simulink model "assignment1DEPRECATED"  (R2023b)
settings: Solver=FixedStepAuto  StartTime=0.0  StopTime=5  FixedStep=1e-3  RelTol=1e-3  EnableMultiTasking=on
undefined symbols (not defined in the file): D0, D1, D10, D11, D12, D13, D2, D3, D4, D5, D6, D7, D8, D9, PTA0, PTA1, PTA2, PTB23, PTB9, PTC16, PTC17, PTC2, PTC3, PTC4, PTD0, PTD1, PTD2, PTD3
libraries: frdmk64flib x18, dspstat3 x3
settings Model: PacingRate=2  ExtModeTrigDuration=5  Creator=Nicholas  LastModifiedBy=Nicholas
settings OptimizationCC: EnhancedBackFolding=on  PassReuseOutputArgsAs=Individual arguments  ZeroExternalMemoryAtStartup=off  ZeroInternalMemoryAtStartup=off  MaxStackSize=64  OptimizeBlockOrder=speed  DifferentSizesBufferReuse=on  OptimizationCustomize=off  EfficientTunableParamExpr=on
settings DebuggingCC: ParameterTunabilityLossMsg=error
settings HardwareCC: ProdBitPerPointer=32  ProdBitPerSizeT=32  ProdBitPerPtrDiffT=32  ProdLargestAtomicInteger=Long  ProdLargestAtomicFloat=Double  ProdWordSize=32  ProdHWDeviceType=ARM Compatible->ARM Cortex
settings SFSimCC: MATLABDynamicMemAlloc=off
settings RTWCC: Description=Embedded Coder  SystemTargetFile=ert.tlc  HardwareBoard=NXP FRDM-K64F  TLCOptions="-aInlineSetEventsForThisBaseRateFcn=TLC_FALSE -aSuppressMultiTaskScheduler=TLC_FALSE  -aRateBasedStepFcn=0"  TemplateMakefile=ert_default_tmf  Toolchain=GNU Tools for ARM Embedded Processors
settings CodeAppCC: ForceParamTrailComments=on  IgnoreCustomStorageClasses=off  OperatorAnnotations=on  SimulinkDataObjDesc=on  SFDataObjDesc=on  InsertBlockDesc=on
settings ERTTargetCC: ExtModeTransport=4  ExtModeMexFile=sendToCommService

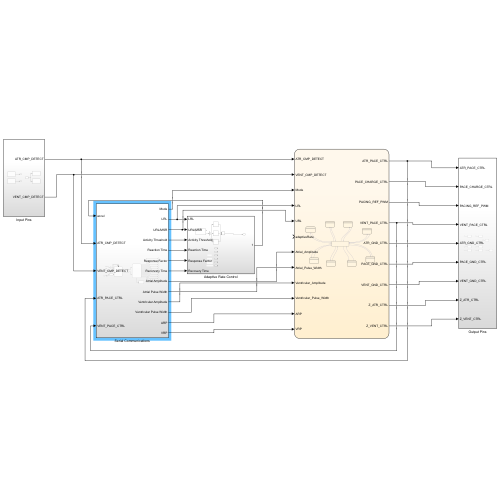
[thumbnail: Simulink's stored preview of the top-level diagram]
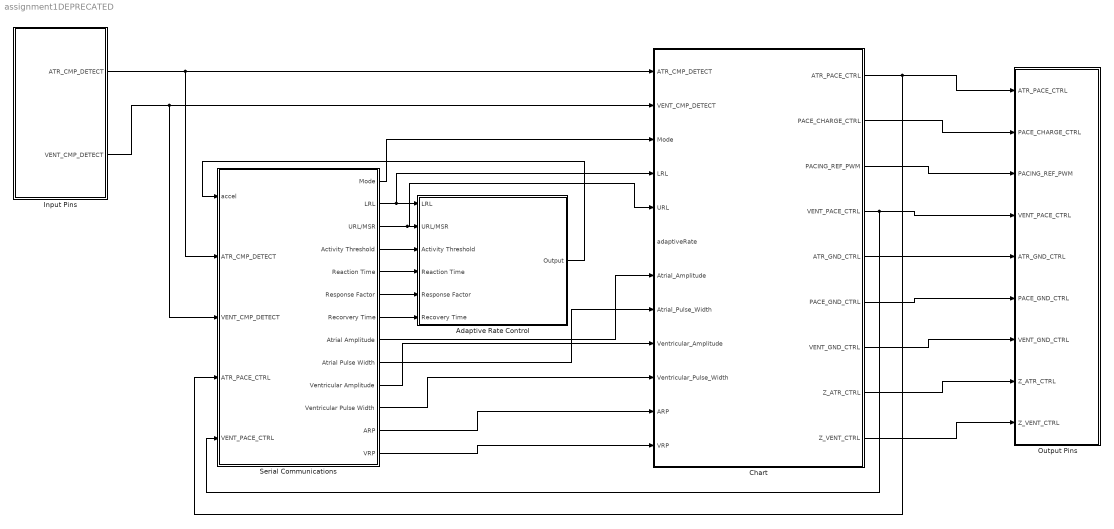
== system assignment1DEPRECATED ==
  Adaptive Rate Control : Subsystem
  Chart : Stateflow chart  TreatAsAtomicUnit=on
      settings: PortSchema="{\"entries\":[{\"content\":{\"sides\":[{\"content\":{\"connectorIds\":[\"In1\",\"In2\",\"In3\",\"In11\",\"In10\",\"In12\",\"In4\",\"In5\",\"In6\",\"In7\",\"In8\",\"In9\"]},\"type\":\"ConnectorPlacement.EquallySpacedRectSide\",\"uuid\":\"f4000909-515d-4a0d-a478-4ca4207159b3\"},{\"content\":{\"connectorIds\":[\"Out1\",\"Out2\",\"Out3\",\"Out4\",\"Out5\",\"Out6\",\"Out7\",\"Out8\",\"Out9\"],\"side\":\"RIGHT\"},\"type\":\"ConnectorPlacement.EquallySpacedRectSide\",\"uuid\":\"74c20bfd-42d0-453a-b20e-355357afff28\"},{\"content\":{\"side\":\"TOP\"},\"type\":\"ConnectorPlacement.EquallySpacedRectSide\",\"uuid\":\"0265984b-474f-4dc0-b8ea-569a4f78f123\"}]},\"type\":\"ConnectorPlacement.EquallySpacedConnector\",\"uuid\":\"44478604-183f-4c3e-8da1-5539e792ac80\"}],\"packageUris\":[\"http://schema.mathworks.com/mf0/Connector/R2020b\"],\"version\":\"1.0\"}"
  Input Pins : Subsystem  Description=Maps the digital and analog input pins of the K64F to named variables as defined in Pacemaker Shield Explained
  Output Pins : Subsystem
  Serial Communications : Subsystem
  wires:
  Input Pins/1(ATR_CMP_DETECT) -> Serial Communications/2(ATR_CMP_DETECT), Chart/1(ATR_CMP_DETECT)
  Input Pins/2(VENT_CMP_DETECT) -> Serial Communications/3(VENT_CMP_DETECT), Chart/2(VENT_CMP_DETECT)
  Chart/9(Z_VENT_CTRL) -> Output Pins/9(Z_VENT_CTRL)
  Chart/4(VENT_PACE_CTRL) -> Serial Communications/5(VENT_PACE_CTRL), Output Pins/4(VENT_PACE_CTRL)
  Chart/8(Z_ATR_CTRL) -> Output Pins/8(Z_ATR_CTRL)
  Chart/3(PACING_REF_PWM) -> Output Pins/3(PACING_REF_PWM)
  Chart/1(ATR_PACE_CTRL) -> Serial Communications/4(ATR_PACE_CTRL), Output Pins/1(ATR_PACE_CTRL)
  Chart/2(PACE_CHARGE_CTRL) -> Output Pins/2(PACE_CHARGE_CTRL)
  Chart/6(PACE_GND_CTRL) -> Output Pins/6(PACE_GND_CTRL)
  Chart/5(ATR_GND_CTRL) -> Output Pins/5(ATR_GND_CTRL)
  Chart/7(VENT_GND_CTRL) -> Output Pins/7(VENT_GND_CTRL)
  Serial Communications/3(URL/MSR) -> Chart/10(URL), Adaptive Rate Control/2(URL/MSR)
  Serial Communications/2(LRL) -> Chart/11(LRL), Adaptive Rate Control/1(LRL)
  Serial Communications/1(Mode) -> Chart/3(Mode)
  Serial Communications/8(Atrial Amplitude) -> Chart/4(Atrial_Amplitude)
  Serial Communications/10(Ventricular Amplitude) -> Chart/6(Ventricular_Amplitude)
  Serial Communications/9(Atrial Pulse Width) -> Chart/5(Atrial_Pulse_Width)
  Serial Communications/11(Ventricular Pulse Width) -> Chart/7(Ventricular_Pulse_Width)
  Serial Communications/13(VRP) -> Chart/9(VRP)
  Serial Communications/12(ARP) -> Chart/8(ARP)
  Adaptive Rate Control/1(Output) -> Serial Communications/1(accel)
  Serial Communications/4(Activity Threshold) -> Adaptive Rate Control/3(Activity Threshold)
  Serial Communications/6(Response Factor) -> Adaptive Rate Control/5(Response Factor)
  Serial Communications/5(Reaction Time) -> Adaptive Rate Control/4(Reaction Time)
  Serial Communications/7(Recorvery Time) -> Adaptive Rate Control/6(Recovery Time)

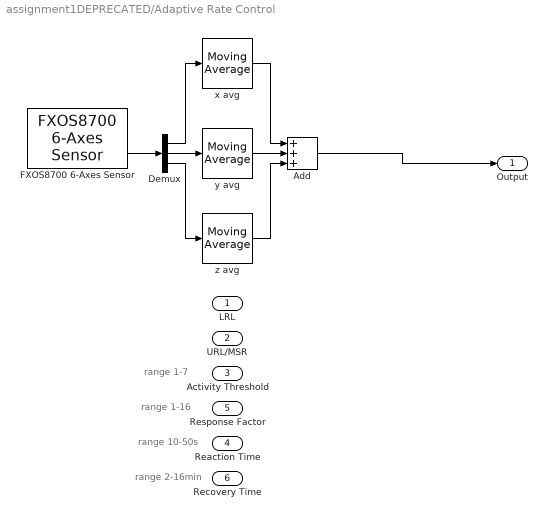
== system assignment1DEPRECATED/Adaptive Rate Control ==
  note: range 2-16min
  note: range 1-16
  note: range 10-50s
  note: range 1-7
  LRL : Inport
  URL/MSR : Inport  Port=2
  Activity Threshold : Inport  Port=3
  Reaction Time : Inport  Port=4
  Response Factor : Inport  Port=5
  Recovery Time : Inport  Port=6
  Add : Sum  Inputs=+++
  Demux : Demux  Outputs=3
  FXOS8700 6-Axes Sensor : frdmk64flib/FXOS8700 6-Axes Sensor  Activesensor=Accelerometer and Magnetometer  ODR=100Hz  HybridODR=400Hz  Accelfullrange=-4g to +4g  SampleTime=-1
  x avg : dspstat3/Moving Average  Method=Sliding window  ForgettingFactorPort=off  SpecifyWindowLength=on  WindowLength=4  OverlapLength=3  AllowArbitraryInputLength=off  ForgettingFactor=0.9  SimulateUsing=Code generation
  y avg : dspstat3/Moving Average  Method=Sliding window  ForgettingFactorPort=off  SpecifyWindowLength=on  WindowLength=4  OverlapLength=3  AllowArbitraryInputLength=off  ForgettingFactor=0.9  SimulateUsing=Code generation
  z avg : dspstat3/Moving Average  Method=Sliding window  ForgettingFactorPort=off  SpecifyWindowLength=on  WindowLength=4  OverlapLength=3  AllowArbitraryInputLength=off  ForgettingFactor=0.9  SimulateUsing=Code generation
  Output : Outport
  wires:
  FXOS8700 6-Axes Sensor/2 -> Demux/1
  Demux/1 -> x avg/1
  Demux/2 -> y avg/1
  Demux/3 -> z avg/1
  x avg/1 -> Add/1
  y avg/1 -> Add/2
  z avg/1 -> Add/3
  Add/1 -> Output/1

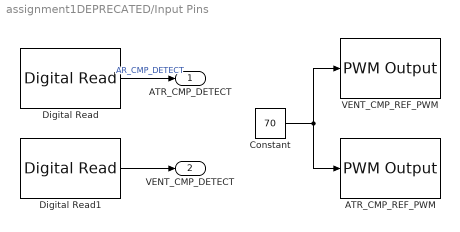
== system assignment1DEPRECATED/Input Pins ==
  ATR_CMP_REF_PWM : frdmk64flib/PWM Output  Whichpin=PTC2 (D6)  InitialFrequency=2000  InitialDutyCycle=0
  Constant : Constant  Value=70
  Digital Read : frdmk64flib/Digital Read  Whichpin=PTC16 (D0)  SampleTime=-1
  Digital Read1 : frdmk64flib/Digital Read  Whichpin=PTC17 (D1)  SampleTime=-1
  VENT_CMP_REF_PWM : frdmk64flib/PWM Output  Whichpin=PTA1 (D3)  InitialFrequency=2000  InitialDutyCycle=0
  ATR_CMP_DETECT : Outport
  VENT_CMP_DETECT : Outport  Port=2
  wires:
  Digital Read1/1 -> VENT_CMP_DETECT/1
  Digital Read/1 -> ATR_CMP_DETECT/1  "AR_CMP_DETECT"
  Constant/1 -> ATR_CMP_REF_PWM/1, VENT_CMP_REF_PWM/1

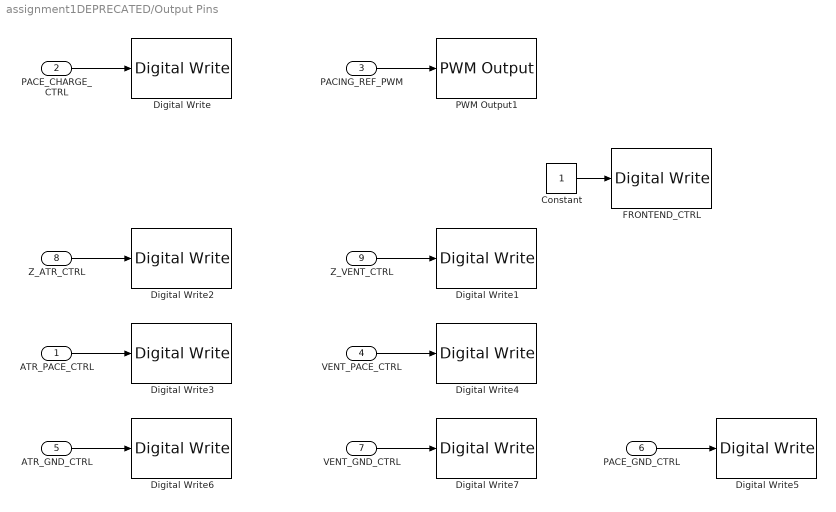
== system assignment1DEPRECATED/Output Pins ==
  ATR_PACE_CTRL : Inport
  PACE_CHARGE_CTRL : Inport  Port=2
  PACING_REF_PWM : Inport  Port=3
  VENT_PACE_CTRL : Inport  Port=4
  ATR_GND_CTRL : Inport  Port=5
  PACE_GND_CTRL : Inport  Port=6
  VENT_GND_CTRL : Inport  Port=7
  Z_ATR_CTRL : Inport  Port=8
  Z_VENT_CTRL : Inport  Port=9
  Constant : Constant
  Digital Write : frdmk64flib/Digital Write  Whichpin=PTB9 (D2)
  Digital Write1 : frdmk64flib/Digital Write  Whichpin=PTC3 (D7)
  Digital Write2 : frdmk64flib/Digital Write  Whichpin=PTB23 (D4)
  Digital Write3 : frdmk64flib/Digital Write  Whichpin=PTA0 (D8)
  Digital Write4 : frdmk64flib/Digital Write  Whichpin=PTC4 (D9)
  Digital Write5 : frdmk64flib/Digital Write  Whichpin=PTD0 (D10)
  Digital Write6 : frdmk64flib/Digital Write  Whichpin=PTD2 (D11)
  Digital Write7 : frdmk64flib/Digital Write  Whichpin=PTD3 (D12)
  FRONTEND_CTRL : frdmk64flib/Digital Write  Whichpin=PTD1 (D13)
  PWM Output1 : frdmk64flib/PWM Output  Whichpin=PTA2 (D5)  InitialFrequency=2000  InitialDutyCycle=0
  wires:
  PACE_CHARGE_CTRL/1 -> Digital Write/1
  Z_ATR_CTRL/1 -> Digital Write2/1
  PACING_REF_PWM/1 -> PWM Output1/1
  Z_VENT_CTRL/1 -> Digital Write1/1
  ATR_PACE_CTRL/1 -> Digital Write3/1
  VENT_PACE_CTRL/1 -> Digital Write4/1
  PACE_GND_CTRL/1 -> Digital Write5/1
  ATR_GND_CTRL/1 -> Digital Write6/1
  VENT_GND_CTRL/1 -> Digital Write7/1
  Constant/1 -> FRONTEND_CTRL/1

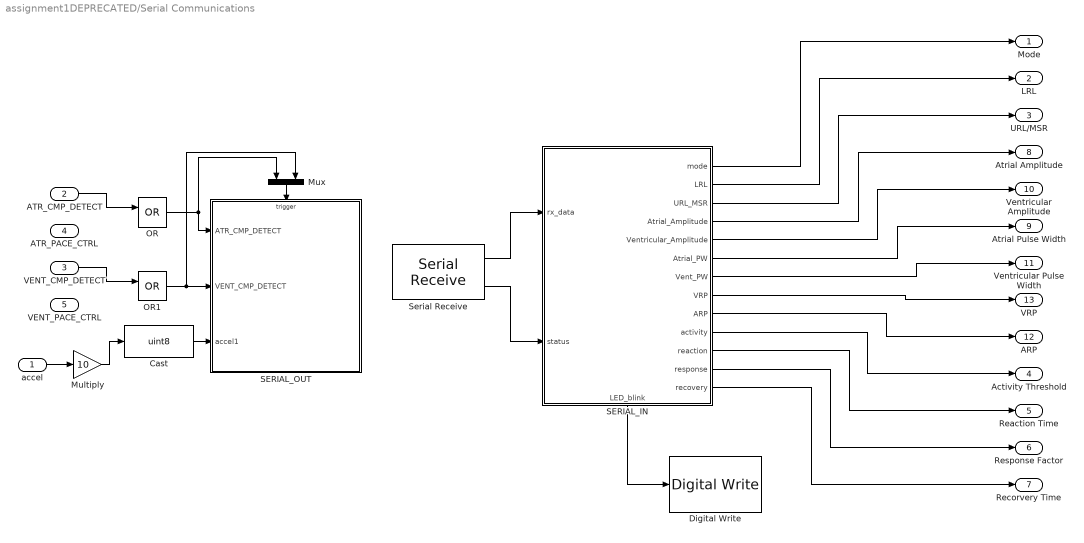
== system assignment1DEPRECATED/Serial Communications ==
  accel : Inport
  ATR_CMP_DETECT : Inport  Port=2
  VENT_CMP_DETECT : Inport  Port=3
  ATR_PACE_CTRL : Inport  Port=4
  VENT_PACE_CTRL : Inport  Port=5
  Cast : DataTypeConversion  OutDataTypeStr=uint8  SaturateOnIntegerOverflow=off  RndMeth=Floor
  Digital Write : frdmk64flib/Digital Write  Whichpin=RED_LED
  Multiply : Gain  Gain=10
  Mux : Mux  Inputs=2
  OR : Logic  Operator=OR  IconShape=distinctive  AllPortsSameDT=off  OutDataTypeStr=boolean
  OR1 : Logic  Operator=OR  IconShape=distinctive  AllPortsSameDT=off  OutDataTypeStr=boolean
  SERIAL_IN : Stateflow chart  TreatAsAtomicUnit=on
      settings: PortSchema="{\"entries\":[{\"content\":{\"sides\":[{\"content\":{\"connectorIds\":[\"In1\",\"In2\"]},\"type\":\"ConnectorPlacement.EquallySpacedRectSide\",\"uuid\":\"ebf63f13-cff1-4dfd-8253-a37fed9b5330\"},{\"content\":{\"connectorIds\":[\"Out1\",\"Out3\",\"Out2\",\"Out5\",\"Out13\",\"Out4\",\"Out7\",\"Out8\",\"Out6\",\"Out9\",\"Out10\",\"Out12\",\"Out11\"],\"side\":\"RIGHT\"},\"type\":\"ConnectorPlacement.EquallySpacedRectSide\",\"uuid\":\"8941ae37-13b3-448c-8772-44937e4639cd\"},{\"content\":{\"side\":\"TOP\"},\"type\":\"ConnectorPlacement.EquallySpacedRectSide\",\"uuid\":\"7a479970-9298-4bcf-8741-da85a2b03343\"},{\"content\":{\"connectorIds\":[\"Out14\"],\"side\":\"BOTTOM\"},\"type\":\"ConnectorPlacement.EquallySpacedRectSide\",\"uuid\":\"dbdb6486-bc4b-4aff-855d-c7d246fcadd5\"}]},\"type\":\"ConnectorPlacement.EquallySpacedConnector\",\"uuid\":\"673a7430-fbb7-42ed-bf30-7a03e16fbc4d\"}],\"packageUris\":[\"http://schema.mathworks.com/mf0/Connector/R2020b\"],\"version\":\"1.0\"}"
  SERIAL_OUT : Subsystem
  Serial Receive : frdmk64flib/Serial Receive  SCIModule=0  Baudrate=uint32(9600)  Parity=None  StopBits=1  HardwareFlowControl=None  ByteOrder=LittleEndian  DataType=uint8  DataLength=16  BlockingMode=off  OutputStatus=on  SampleTime=-1
  Mode : Outport
  LRL : Outport  Port=2
  URL/MSR : Outport  Port=3
  Activity Threshold : Outport  Port=4
  Reaction Time : Outport  Port=5
  Response Factor : Outport  Port=6
  Recorvery Time : Outport  Port=7
  Atrial Amplitude : Outport  Port=8
  Atrial Pulse Width : Outport  Port=9
  Ventricular Amplitude : Outport  Port=10
  Ventricular Pulse Width : Outport  Port=11
  ARP : Outport  Port=12
  VRP : Outport  Port=13
  wires:
  Serial Receive/2 -> SERIAL_IN/2(status)
  Serial Receive/1 -> SERIAL_IN/1(rx_data)
  SERIAL_IN/1(mode) -> Mode/1
  SERIAL_IN/3(LRL) -> LRL/1
  SERIAL_IN/2(URL_MSR) -> URL/MSR/1
  SERIAL_IN/5(Atrial_Amplitude) -> Atrial Amplitude/1
  SERIAL_IN/4(Atrial_PW) -> Atrial Pulse Width/1
  SERIAL_IN/6(ARP) -> ARP/1
  SERIAL_IN/7(Vent_PW) -> Ventricular Pulse Width/1
  SERIAL_IN/8(VRP) -> VRP/1
  SERIAL_IN/9(activity) -> Activity Threshold/1
  SERIAL_IN/10(reaction) -> Reaction Time/1
  SERIAL_IN/11(recovery) -> Recorvery Time/1
  SERIAL_IN/12(response) -> Response Factor/1
  SERIAL_IN/13(Ventricular_Amplitude) -> Ventricular Amplitude/1
  Mux/1 -> SERIAL_OUT/Trigger
  accel/1 -> Multiply/1
  ATR_CMP_DETECT/1 -> OR/1
  VENT_CMP_DETECT/1 -> OR1/1
  OR/1 -> SERIAL_OUT/1(ATR_CMP_DETECT), Mux/1
  OR1/1 -> SERIAL_OUT/2(VENT_CMP_DETECT), Mux/2
  SERIAL_IN/14(LED_blink) -> Digital Write/1
  Multiply/1 -> Cast/1
  Cast/1 -> SERIAL_OUT/3(accel1)

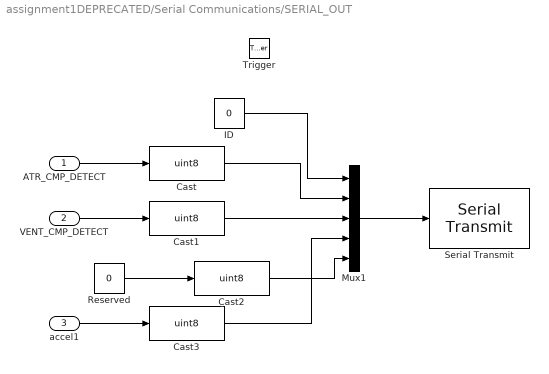
== system assignment1DEPRECATED/Serial Communications/SERIAL_OUT ==
  ATR_CMP_DETECT : Inport
  VENT_CMP_DETECT : Inport  Port=2
  accel1 : Inport  Port=3
  Trigger : TriggerPort  VariantControl=(inherit)  PortDimensions=1
  Cast{,1..3} (4 alike) : DataTypeConversion  OutDataTypeStr=uint8  SaturateOnIntegerOverflow=off  RndMeth=Floor
  ID : Constant  Value=0  OutDataTypeStr=uint8
  Mux1 : Mux  Inputs=5
  Reserved : Constant  Value=0
  Serial Transmit : frdmk64flib/Serial Transmit  SCIModule=0  Baudrate=uint32(9600)  Parity=None  StopBits=1  HardwareFlowControl=None  ByteOrder=LittleEndian  BlockingMode=on  OutputStatus=off
  wires:
  VENT_CMP_DETECT/1 -> Cast1/1
  Cast1/1 -> Mux1/3
  Cast3/1 -> Mux1/4
  Cast/1 -> Mux1/2
  accel1/1 -> Cast3/1
  ID/1 -> Mux1/1
  Reserved/1 -> Cast2/1
  Mux1/1 -> Serial Transmit/1
  ATR_CMP_DETECT/1 -> Cast/1
  Cast2/1 -> Mux1/5

== stateflow chart assignment1DEPRECATED/Serial Communications/SERIAL_IN ==
  state success
    entry:
    LED_blink = 1;
    mode = rx_data(1);
    LRL = rx_data(2);
    URL_MSR = rx_data(3);
    Atrial_Amplitude = double(rx_data(4)/10);
    Ventricular_Amplitude = double(rx_data(5)/10);
    Atrial_PW = rx_data(6);
    Vent_PW = rx_data(7);
    VRP = uint32(rx_data(8)*10);
    ARP = uint32(rx_data(9)*10);
    activity = rx_data(10);
    reaction = rx_data(11);
    response = rx_data(12);
    recovery = rx_data(13);
  state Initial
    entry:
    mode = 255;
  state standby
    entry:
    LED_blink = 0;
  (default) -> Initial
  success -> standby : [et(sec) >= 1]
  standby -> success : [status == 0]
  Initial -> standby
  data: rx_data input; status input; mode output uint8; URL_MSR output; LRL output; Atrial_PW output; Atrial_Amplitude output double; ARP output uint32; Vent_PW output; VRP output uint32; activity output; reaction output; recovery output; response output; Ventricular_Amplitude output double; LED_blink output

== stateflow chart assignment1DEPRECATED/Chart ==
  state VOO
    state setup
      entry:
      ventDutyCycle = (Ventricular_Amplitude/5)*100
      ventWait = single(Rate_ms - Ventricular_Pulse_Width)
    state charge_discharge
      entry:
      %discharge c21
      PACE_GND_CTRL = 0
      VENT_PACE_CTRL = 0
      Z_ATR_CTRL = 0
      Z_VENT_CTRL = 0
      ATR_PACE_CTRL = 0
      ATR_GND_CTRL = 0
      VENT_GND_CTRL = 1
      %charge c22
      VENT_PACE_CTRL = 0
      ATR_PACE_CTRL = 0
      PACING_REF_PWM = double(ventDutyCycle)
      PACE_CHARGE_CTRL = 1
    state pace
      PACE_CHARGE_CTRL = 0
      PACE_GND_CTRL = 1
      ATR_PACE_CTRL = 0
      ATR_GND_CTRL = 0
      Z_ATR_CTRL = 0
      Z_VENT_CTRL = 0
      VENT_GND_CTRL = 0
      VENT_PACE_CTRL = 1
    (default) -> VOO.setup
    VOO.setup -> VOO.charge_discharge
    VOO.charge_discharge -> VOO.pace : [et(msec) >= ventWait]
    VOO.pace -> VOO.charge_discharge : [et(msec) >= Ventricular_Pulse_Width]
  state AAI
    state setup
      entry:
      atrialDutyCycle = (Atrial_Amplitude/5)*100
      atrWait = single(Rate_ms - Atrial_Pulse_Width)
      timeToPace = atrWait
    state refractory_period
    state charge_discharge_EN
      entry:
      %discharge c21
      PACE_GND_CTRL = 0
      ATR_PACE_CTRL = 0
      Z_ATR_CTRL = 0
      Z_VENT_CTRL = 0
      VENT_PACE_CTRL = 0
      VENT_GND_CTRL = 0
      ATR_GND_CTRL = 1
      %charge c22
      ATR_PACE_CTRL = 0
      VENT_PACE_CTRL = 0
      PACING_REF_PWM = atrialDutyCycle
      PACE_CHARGE_CTRL = 1
    state sense_wait
      exit:
      timeToPace = timeToPace - et(msec)
    state pace
      entry:
      PACE_CHARGE_CTRL = 0
      PACE_GND_CTRL = 1
      VENT_PACE_CTRL = 0
      VENT_GND_CTRL = 0
      Z_ATR_CTRL = 0
      Z_VENT_CTRL = 0
      ATR_GND_CTRL = 0
      ATR_PACE_CTRL = 1
      %reset timer
      timeToPace = atrWait
    (default) -> AAI.setup
    AAI.setup -> AAI.charge_discharge_EN
    AAI.refractory_period -> AAI.sense_wait : [et(msec) >= ARP]
    AAI.sense_wait -> AAI.refractory_period [order 1] : [ATR_CMP_DETECT == 1]
    AAI.charge_discharge_EN -> AAI.sense_wait
    AAI.sense_wait -> AAI.pace [order 2] : [et(msec) >= timeToPace]
    AAI.pace -> AAI.charge_discharge_EN : [et(msec) >= Atrial_Pulse_Width]
  state AOO
    state setup
      entry:
      atrialDutyCycle = (Atrial_Amplitude/5)*100
      atrWait = single(Rate_ms - Atrial_Pulse_Width)
    state charge_discharge
      entry:
      %discharge c21
      PACE_GND_CTRL = 0
      ATR_PACE_CTRL = 0
      Z_ATR_CTRL = 0
      Z_VENT_CTRL = 0
      VENT_PACE_CTRL = 0
      VENT_GND_CTRL = 0
      ATR_GND_CTRL = 1
      %charge c22
      ATR_PACE_CTRL = 0
      VENT_PACE_CTRL = 0
      PACING_REF_PWM = atrialDutyCycle
      PACE_CHARGE_CTRL = 1
    state pace
      PACE_CHARGE_CTRL = 0
      PACE_GND_CTRL = 1
      VENT_PACE_CTRL = 0
      VENT_GND_CTRL = 0
      Z_ATR_CTRL = 0
      Z_VENT_CTRL = 0
      ATR_GND_CTRL = 0
      ATR_PACE_CTRL = 1
    (default) -> AOO.setup
    AOO.setup -> AOO.charge_discharge
    AOO.charge_discharge -> AOO.pace : [et(msec) >= atrWait]
    AOO.pace -> AOO.charge_discharge : [et(msec) >= Atrial_Pulse_Width]
  state VVI
    state setup
      entry:
      ventDutyCycle = (Ventricular_Amplitude/5)*100
      ventWait = single(Rate_ms - Ventricular_Pulse_Width)
    state charge_discharge_EN
      entry:
      %discharge c21
      PACE_GND_CTRL = 0
      VENT_PACE_CTRL = 0
      Z_VENT_CTRL = 0
      Z_ATR_CTRL = 0
      ATR_PACE_CTRL = 0
      ATR_GND_CTRL = 0
      VENT_GND_CTRL = 1
      %charge c22
      VENT_PACE_CTRL = 0
      ATR_PACE_CTRL = 0
      PACING_REF_PWM = double(ventDutyCycle)
      PACE_CHARGE_CTRL = 1
    state refractory
      %do nothing
      %after a pace
    state sense_wait
      %check for new
      %nat pace
    state pace
      entry:
      PACE_CHARGE_CTRL = 0
      PACE_GND_CTRL = 1
      ATR_PACE_CTRL = 0
      ATR_GND_CTRL = 0
      Z_VENT_CTRL = 0
      Z_ATR_CTRL = 0
      VENT_GND_CTRL = 0
      VENT_PACE_CTRL = 1
    (default) -> VVI.setup
    VVI.setup -> VVI.charge_discharge_EN
    VVI.sense_wait -> refractory [order 2] : [VENT_CMP_DETECT == 1]
    VVI.charge_discharge_EN -> refractory
    refractory -> VVI.sense_wait : [et(msec) >= VRP]
    VVI.sense_wait -> VVI.pace [order 1] : [et(msec) >= ventWait - double(VRP)]
    VVI.pace -> VVI.charge_discharge_EN : [et(msec) >= Ventricular_Pulse_Width]
  state Start
    entry:
    Rate_ms = double(1000/(LRL/60))
  state VVIR
    state setup
      entry:
      ventDutyCycle = (Ventricular_Amplitude/5)*100
    state refractory_period
    state charge_discharge_EN
      entry:
      %set new rate
      Rate_ms = 1000/(adaptiveRate/60)
      atrWait = single(Rate_ms - Atrial_Pulse_Width)
      timeToPace = ventWait
      %discharge c21
      PACE_GND_CTRL = 0
      VENT_PACE_CTRL = 0
      Z_VENT_CTRL = 0
      Z_ATR_CTRL = 0
      ATR_PACE_CTRL = 0
      ATR_GND_CTRL = 0
      VENT_GND_CTRL = 1
      %charge c22
      VENT_PACE_CTRL = 0
      ATR_PACE_CTRL = 0
      PACING_REF_PWM = double(ventDutyCycle)
      PACE_CHARGE_CTRL = 1
    state sense_wait
      exit:
      timeToPace = timeToPace - et(msec)
    state pace
      entry:
      PACE_CHARGE_CTRL = 0
      PACE_GND_CTRL = 1
      ATR_PACE_CTRL = 0
      ATR_GND_CTRL = 0
      Z_VENT_CTRL = 0
      Z_ATR_CTRL = 0
      VENT_GND_CTRL = 0
      VENT_PACE_CTRL = 1
      %reset timer
      timeToPace = ventWait
    (default) -> VVIR.setup
    VVIR.setup -> VVIR.charge_discharge_EN
    VVIR.refractory_period -> VVIR.sense_wait : [et(msec) >= VRP]
    VVIR.sense_wait -> VVIR.refractory_period [order 1] : [VENT_CMP_DETECT == 1]
    VVIR.charge_discharge_EN -> VVIR.sense_wait
    VVIR.sense_wait -> VVIR.pace [order 2] : [et(msec) >= timeToPace]
    VVIR.pace -> VVIR.charge_discharge_EN : [et(msec) >= Ventricular_Pulse_Width]
  state AOOR
    state setup
      entry:
      atrialDutyCycle = (Atrial_Amplitude/5)*100
    state charge_discharge
      entry:
      %set new rate
      Rate_ms = 1000/(adaptiveRate/60)
      atrWait = single(Rate_ms - Atrial_Pulse_Width)
      %discharge c21
      PACE_GND_CTRL = 0
      ATR_PACE_CTRL = 0
      Z_ATR_CTRL = 0
      Z_VENT_CTRL = 0
      VENT_PACE_CTRL = 0
      VENT_GND_CTRL = 0
      ATR_GND_CTRL = 1
      %charge c22
      ATR_PACE_CTRL = 0
      VENT_PACE_CTRL = 0
      PACING_REF_PWM = atrialDutyCycle
      PACE_CHARGE_CTRL = 1
    state pace
      PACE_CHARGE_CTRL = 0
      PACE_GND_CTRL = 1
      VENT_PACE_CTRL = 0
      VENT_GND_CTRL = 0
      Z_ATR_CTRL = 0
      Z_VENT_CTRL = 0
      ATR_GND_CTRL = 0
      ATR_PACE_CTRL = 1
    (default) -> AOOR.setup
    AOOR.setup -> AOOR.charge_discharge
    AOOR.charge_discharge -> AOOR.pace : [et(msec) >= atrWait]
    AOOR.pace -> AOOR.charge_discharge : [et(msec) >= Atrial_Pulse_Width]
  state VOOR
    state setup
      entry:
      ventDutyCycle = (Ventricular_Amplitude/5)*100
    state charge_discharge
      entry:
      %set new rate
      Rate_ms = 1000/(adaptiveRate/60)
      ventWait = single(Rate_ms - Ventricular_Pulse_Width)
      %discharge c21
      PACE_GND_CTRL = 0
      VENT_PACE_CTRL = 0
      Z_ATR_CTRL = 0
      Z_VENT_CTRL = 0
      ATR_PACE_CTRL = 0
      ATR_GND_CTRL = 0
      VENT_GND_CTRL = 1
      %charge c22
      VENT_PACE_CTRL = 0
      ATR_PACE_CTRL = 0
      PACING_REF_PWM = double(ventDutyCycle)
      PACE_CHARGE_CTRL = 1
    state pace
      PACE_CHARGE_CTRL = 0
      PACE_GND_CTRL = 1
      ATR_PACE_CTRL = 0
      ATR_GND_CTRL = 0
      Z_ATR_CTRL = 0
      Z_VENT_CTRL = 0
      VENT_GND_CTRL = 0
      VENT_PACE_CTRL = 1
    (default) -> VOOR.setup
    VOOR.setup -> VOOR.charge_discharge
    VOOR.charge_discharge -> VOOR.pace : [et(msec) >= ventWait]
    VOOR.pace -> VOOR.charge_discharge : [et(msec) >= Ventricular_Pulse_Width]
  state AAIR
    state setup
      entry:
      atrialDutyCycle = (Atrial_Amplitude/5)*100
    state refractory_period
    state charge_discharge_EN
      entry:
      %set new rate
      Rate_ms = 1000/(adaptiveRate/60)
      atrWait = single(Rate_ms - Atrial_Pulse_Width)
      timeToPace = atrWait
      %discharge c21
      PACE_GND_CTRL = 0
      ATR_PACE_CTRL = 0
      Z_ATR_CTRL = 0
      Z_VENT_CTRL = 0
      VENT_PACE_CTRL = 0
      VENT_GND_CTRL = 0
      ATR_GND_CTRL = 1
      %charge c22
      ATR_PACE_CTRL = 0
      VENT_PACE_CTRL = 0
      PACING_REF_PWM = atrialDutyCycle
      PACE_CHARGE_CTRL = 1
    state sense_wait
      exit:
      timeToPace = timeToPace - et(msec)
    state pace
      entry:
      PACE_CHARGE_CTRL = 0
      PACE_GND_CTRL = 1
      VENT_PACE_CTRL = 0
      VENT_GND_CTRL = 0
      Z_ATR_CTRL = 0
      Z_VENT_CTRL = 0
      ATR_GND_CTRL = 0
      ATR_PACE_CTRL = 1
      %reset timer
      timeToPace = atrWait
    (default) -> AAIR.setup
    AAIR.setup -> AAIR.charge_discharge_EN
    AAIR.refractory_period -> AAIR.sense_wait : [et(msec) >= ARP]
    AAIR.sense_wait -> AAIR.refractory_period [order 1] : [ATR_CMP_DETECT == 1]
    AAIR.charge_discharge_EN -> AAIR.sense_wait
    AAIR.sense_wait -> AAIR.pace [order 2] : [et(msec) >= timeToPace]
    AAIR.pace -> AAIR.charge_discharge_EN : [et(msec) >= Atrial_Pulse_Width]
  Start -> VOO [order 2] : [Mode == 1]
  VOO -> Start : [Mode ~= 1]
  Start -> AAI [order 4] : [Mode == 2]
  AAI -> Start : [Mode ~= 2]
  Start -> AOO [order 1] : [Mode == 0]
  AOO -> Start : [Mode ~= 0]
  Start -> VVI [order 3] : [Mode == 3]
  VVI -> Start : [Mode ~= 3]
  (default) -> Start
  VVIR -> Start : [Mode ~= 7]
  Start -> AOOR [order 5] : [Mode == 4]
  Start -> VVIR [order 8] : [Mode == 7]
  AOOR -> Start : [Mode ~= 4]
  Start -> VOOR [order 6] : [Mode == 5]
  VOOR -> Start : [Mode ~= 5]
  Start -> AAIR [order 7] : [Mode == 6]
  AAIR -> Start : [Mode ~= 6]
  data: ATR_CMP_DETECT input boolean; VENT_CMP_DETECT input boolean; Mode input uint8 [0..4]; Atrial_Amplitude input double; Atrial_Pulse_Width input uint8; Ventricular_Amplitude input double; Ventricular_Pulse_Width input uint8; atrialDutyCycle local; Rate_ms local double; atrWait local single; ATR_PACE_CTRL output; PACE_CHARGE_CTRL output; PACING_REF_PWM output; VENT_PACE_CTRL output; ATR_GND_CTRL output; PACE_GND_CTRL output; VENT_GND_CTRL output; Z_ATR_CTRL output; Z_VENT_CTRL output; ventWait local; ventDutyCycle local; ARP input uint32; VRP input uint32; URL input; LRL input; adaptiveRate input double; timeToPace local
